simulink model "prototype_test_simulink"  (R2021a)
settings: Solver=VariableStepAuto  StartTime=0.0  StopTime=10.0  RelTol=1e-3
settings Model: Creator=anlun  LastModifiedBy=anlun

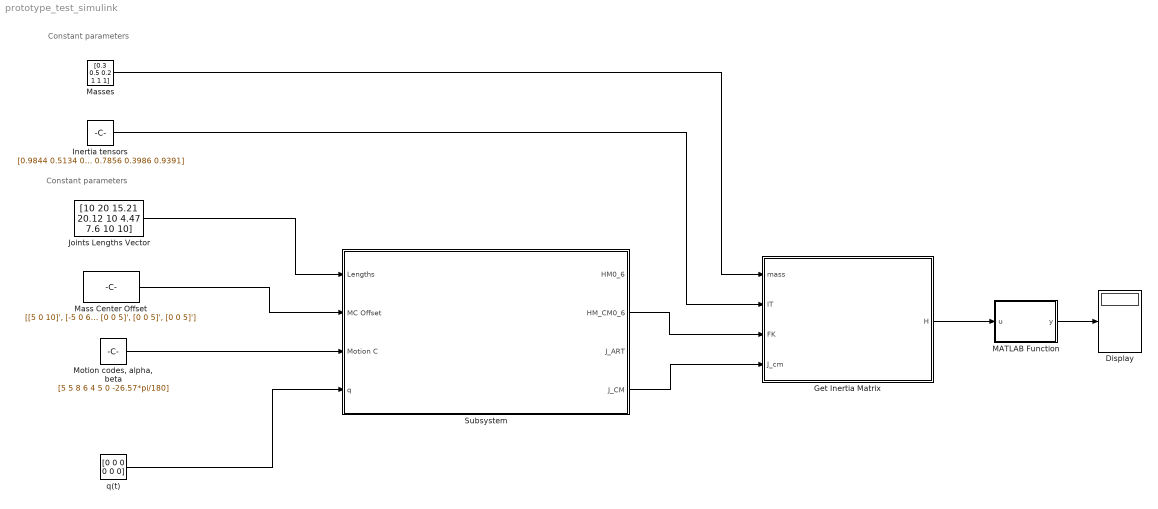
== system prototype_test_simulink ==
  note: Constant parameters
  note: Constant parameters
  Display : Display
  Get Inertia Matrix : MATLAB Function  TreatAsAtomicUnit=on
  Inertia tensors : Constant  Value=|
      | [0.9844 0.5134 0.1339 0.8589 0.1776 0.0309 0.7856 0.3986 0.9391;
      |                    0.9844 0.5134 0.1339 0.8589 0.1776 0.0309 0.7856 0.3986 0.9391;
      |                    0.9844 0.5134 0.1339 0.8589 0.1776 0.0309 0.7856 0.3986 0.9391;
      |                    0.9844 0.5134 0.1339 0.8589 0.1776 0.0309 0.7856 0.3986 0.9391;
      |                    0.9844 0.5134 0.1339 0.8589 0.1776 0.0309 0.7856 0.3986 0.9391;
      |                    0.9844 0.5134 0.1339 0.8589 0.1776 0.0309 0.7856 0.3986 0.9391]
  Joints Lengths Vector : Constant  Value=[10 20 15.21 20.12 10 4.47 7.6 10 10]
  MATLAB Function : MATLAB Function  TreatAsAtomicUnit=on
  Mass Center Offset : Constant  Value=[[5 0 10]', [-5 0 6]', [-3 0 10]', [0 0 5]', [0 0 5]', [0 0 5]']
  Masses : Constant  Value=[0.3 0.5 0.2 1 1 1]
  "Motion codes, alpha, beta" : Constant  Value=[5 5 8 6 4 5 0 -26.57*pi/180]
  Subsystem : Subsystem
  q(t) : Constant  Value=[0 0 0 0 0 0]
  wires:
  Joints Lengths Vector/1 -> Subsystem/1(Lengths)
  Mass Center Offset/1 -> Subsystem/2(MC Offset)
  "Motion codes, alpha, beta"/1 -> Subsystem/3(Motion C)
  q(t)/1 -> Subsystem/4(q)
  MATLAB Function/1(y) -> Display/1
  Masses/1 -> Get Inertia Matrix/1(mass)
  Inertia tensors/1 -> Get Inertia Matrix/2(IT)
  Subsystem/2(HM_CM0_6) -> Get Inertia Matrix/3(FK)
  Subsystem/4(J_CM) -> Get Inertia Matrix/4(J_cm)
  Get Inertia Matrix/1(H) -> MATLAB Function/1(u)

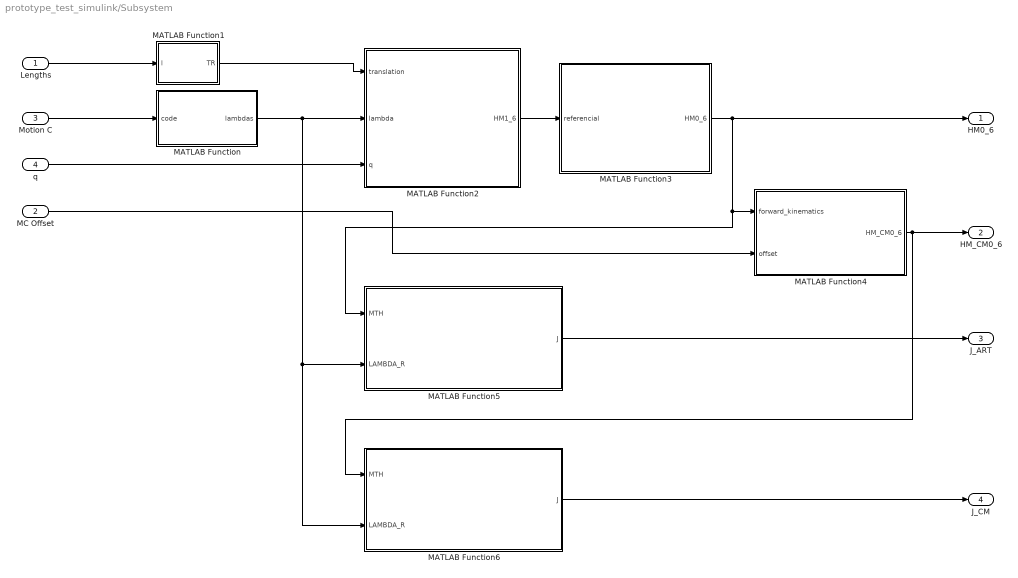
== system prototype_test_simulink/Subsystem ==
  Lengths : Inport
  MC Offset : Inport  Port=2
  Motion C : Inport  Port=3
  q : Inport  Port=4
  MATLAB Function : MATLAB Function  TreatAsAtomicUnit=on
  MATLAB Function1 : MATLAB Function  TreatAsAtomicUnit=on
  MATLAB Function2 : MATLAB Function  TreatAsAtomicUnit=on
  MATLAB Function3 : MATLAB Function  TreatAsAtomicUnit=on
  MATLAB Function4 : MATLAB Function  TreatAsAtomicUnit=on
  MATLAB Function5 : MATLAB Function  TreatAsAtomicUnit=on
  MATLAB Function6 : MATLAB Function  TreatAsAtomicUnit=on
  HM0_6 : Outport
  HM_CM0_6 : Outport  Port=2
  J_ART : Outport  Port=3
  J_CM : Outport  Port=4
  wires:
  Motion C/1 -> MATLAB Function/1(code)
  Lengths/1 -> MATLAB Function1/1(l)
  MATLAB Function1/1(TR) -> MATLAB Function2/1(translation)
  MATLAB Function/1(lambdas) -> MATLAB Function6/2(LAMBDA_R), MATLAB Function5/2(LAMBDA_R), MATLAB Function2/2(lambda)
  q/1 -> MATLAB Function2/3(q)
  MATLAB Function2/1(HM1_6) -> MATLAB Function3/1(referencial)
  MATLAB Function3/1(HM0_6) -> MATLAB Function5/1(MTH), MATLAB Function4/1(forward_kinematics), HM0_6/1
  MC Offset/1 -> MATLAB Function4/2(offset)
  MATLAB Function4/1(HM_CM0_6) -> MATLAB Function6/1(MTH), HM_CM0_6/1
  MATLAB Function5/1(J) -> J_ART/1
  MATLAB Function6/1(J) -> J_CM/1

== matlab function prototype_test_simulink/Subsystem/MATLAB Function1 ==
  data: l input; TR output
function TR = translation_ref(l)
    TR = [[0 0 0]',[l(1) 0 l(2)]',[-l(7) 0 l(3)]',[-l(6) 0 l(4)]',[0 0 l(5)]',[0 0 l(8)]',[0 0 l(9)]'];
end

== matlab function prototype_test_simulink/Subsystem/MATLAB Function ==
  data: code input; lambdas output
function lambdas = rotation_vectors(code)
    a = code(end-1);
    b = code(end);
    lambdas = zeros(3,length(code)-2);
    %lambdas = cell(1,length(code));
    for i = 1:length(code)-2
        switch code(i)
            case 0
                lambda = [0 0 0]';
            case 4
                lambda = [1 0 0]';
            case 5
                lambda = [0 1 0]';
            case 6 
                lambda = [0 0 1]';
            otherwise
                lambda = [cos(a)*sin(b) sin(a)*sin(b) cos(b)]';
        end
        lambdas(:,i) = lambda; 
    end
end

== matlab function prototype_test_simulink/Subsystem/MATLAB Function2 ==
  data: translation input; HM1_6 output; lambda input; q input
function HM1_6 = local_htm(translation, lambda, q) 
    num_ref = length(lambda);
    HM1_6 = zeros(num_ref,16);
    for i = 1:num_ref
        vec = lambda(:,i)*q(i);
        opc = [0 -vec(3) vec(2); vec(3) 0 -vec(1); -vec(2) vec(1) 0];
        rotation_matrix = expm(opc);
        hm_i = [rotation_matrix translation(:,i); 0 0 0 1];
        HM1_6(i,:) = reshape(hm_i,1,16);
    end
end

== matlab function prototype_test_simulink/MATLAB Function ==
  data: u input; y output
function y = fcn(u)
    y = zeros(1,2);
    y(1) = size(u,1);
    y(2) = size(u,2);
end

== matlab function prototype_test_simulink/Subsystem/MATLAB Function3 ==
  data: referencial input; HM0_6 output
function HM0_6 = forward_kmt(referencial)
    num_ref = size(referencial,1);
    HM0_6 = zeros(num_ref, 16);
    HM0_6(1,:) = referencial(1,:);
    for i = 2:num_ref
        ht_prev = reshape(HM0_6(i-1,:),4,4);
        ht_ref = reshape(referencial(i,:),4,4);
        HM0_6(i,:) = reshape(ht_prev*ht_ref,1,16);
    end
end

== matlab function prototype_test_simulink/Subsystem/MATLAB Function4 ==
  data: forward_kinematics input; HM_CM0_6 output; offset input
function HM_CM0_6 = FK_CM(forward_kinematics, offset)
    num_cm = size(offset, 2);
    HM_CM0_6 = zeros(num_cm, 16);
    I = eye(3);
    for i = 1:num_cm
        HM_CM0_i = reshape(forward_kinematics(i,:),4,4)*[I offset(:,i); 0 0 0 1]; 
        HM_CM0_6(i,:) = reshape(HM_CM0_i, 1, 16);
    end
end

== matlab function prototype_test_simulink/Subsystem/MATLAB Function5 ==
  data: MTH input; J output; LAMBDA_R input
function J = jacobian_generator(MTH, LAMBDA_R)
    n = size(LAMBDA_R,2);
    J = zeros(n,(6*n));
    j_w = zeros(3, n);
    for i = 1:n
        j_i = zeros(6, n);
        j_v = zeros(3, n);
        
        mth0_i = reshape(MTH(i,:), 4, 4);
        mth_r_i = mth0_i(1:3,1:3);
        d_p = mth0_i(1:3,4);
        lambda_r_i = LAMBDA_R(:,i);

        %--Jacobiano de velocidad angular--
        j_w_i = mth_r_i*lambda_r_i;
        j_w(:,i) = j_w_i;
        
        %--Jacobiano de velocidad lineal--
        for j = 1:i
            mth0_j = reshape(MTH(j,:), 4, 4);
            d_j = mth0_j(1:3,4);
            j_w_j = j_w(:,j);
            j_v(:,j) = cross(j_w_j, (d_p-d_j));
        end

        j_i(1:3, :) = j_v;
        j_i(4:6, :) = j_w;
        
        J(i,:) = reshape(j_i, 1, (6*n));
    end
end

== matlab function prototype_test_simulink/Subsystem/MATLAB Function6 ==
  data: MTH input; J output; LAMBDA_R input
function J = jacobian_generator(MTH, LAMBDA_R)
    n = size(LAMBDA_R,2);
    J = zeros(n,(6*n));
    j_w = zeros(3, n);
    for i = 1:n
        j_i = zeros(6, n);
        j_v = zeros(3, n);
        
        mth0_i = reshape(MTH(i,:), 4, 4);
        mth_r_i = mth0_i(1:3,1:3);
        d_p = mth0_i(1:3,4);
        lambda_r_i = LAMBDA_R(:,i);

        %--Jacobiano de velocidad angular--
        j_w_i = mth_r_i*lambda_r_i;
        j_w(:,i) = j_w_i;
        
        %--Jacobiano de velocidad lineal--
        for j = 1:i
            mth0_j = reshape(MTH(j,:), 4, 4);
            d_j = mth0_j(1:3,4);
            j_w_j = j_w(:,j);
            j_v(:,j) = cross(j_w_j, (d_p-d_j));
        end

        j_i(1:3, :) = j_v;
        j_i(4:6, :) = j_w;
        
        J(i,:) = reshape(j_i, 1, (6*n));
    end
end

== matlab function prototype_test_simulink/Get Inertia Matrix ==
  data: mass input; IT input; FK input; H output; J_cm input
function H = inertia_matrix(mass, IT, FK, J_cm)
    N = length(mass);
    H = zeros(N);
    for i  = 1:N
        J_cm_i = reshape(J_cm(i,:), 6, N);
        Jv_cm_i = J_cm_i(1:3,:);
        Jw_cm_i = J_cm_i(4:6,:);
        
        FK_i = reshape(FK(i,:), 4, 4);
        IT_i = reshape(IT(i,:), 3, 3);
        
        rotmatrix0_i = FK_i(1:3,1:3);
        linear = mass(i)*(Jv_cm_i)'*Jv_cm_i;
        angular = (Jw_cm_i')*(rotmatrix0_i)*(IT_i)*(rotmatrix0_i')*(Jw_cm_i);
        H = H + linear + angular;
    end
        H = (1/2)*H;
end
